simulink model "rover_sw_pwrtrain_24b"  (R2024b)
settings: Solver=FixedStepAuto  StartTime=0.0  StopTime=inf  FixedStep=.01  RelTol=1e-3
values from neighbouring files (symbols this model uses):
  collision_flt : value not decoded    [rover_param.sldd]
  FALSE = 0.0    [rover_param.sldd]
  TRUE = 1.0    [rover_param.sldd]
undefined symbols (not defined in the file or in its folder): DiscIntNeverNeededParam
libraries: ros2lib x36, simulink x5
settings Model: DataDictionary=rover_param.sldd  Creator=abhijeetsaini  LastModifiedBy=saini
settings OptimizationCC: DefaultParameterBehavior=Inlined  EnhancedBackFolding=on  PassReuseOutputArgsThreshold=0  ZeroExternalMemoryAtStartup=off  ZeroInternalMemoryAtStartup=off  MaxStackSize=64  OptimizeBlockOrder=speed  DifferentSizesBufferReuse=on  OptimizationCustomize=off
settings DebuggingCC: ParameterTunabilityLossMsg=error
settings HardwareCC: ProdBitPerLong=64  ProdHWDeviceType=Apple->ARM64  UseEmbeddedCoderFeatures=off
settings RTWCC: Description=Embedded Coder  SystemTargetFile=ert.tlc  HardwareBoard=Robot Operating System 2 (ROS 2)  TLCOptions="-aInlineSetEventsForThisBaseRateFcn=TLC_FALSE -aSuppressMultiTaskScheduler=TLC_FALSE  -aRateBasedStepFcn=0"  TemplateMakefile=ert_default_tmf  Toolchain=Colcon Tools  TargetLang=C++
settings RTWCC: CustomSourceCode=|
  | int  vesc_open_noargs(void);
  | void vesc_close(void);
  | int  vesc_send_duty(double duty);
  | int  vesc_poll(float* v_in, float* t_mos, float* t_motor);
settings CodeAppCC: ForceParamTrailComments=on  OperatorAnnotations=on
settings ERTTargetCC: ERTCustomFileBanners=off  CodeInterfacePackaging=C++ class  SupportContinuousTime=on  SupportNonInlinedSFcns=on  RemoveResetFunc=off  ModelStepFunctionPrototypeControlCompliant=off  RootIOFormat=Structure reference

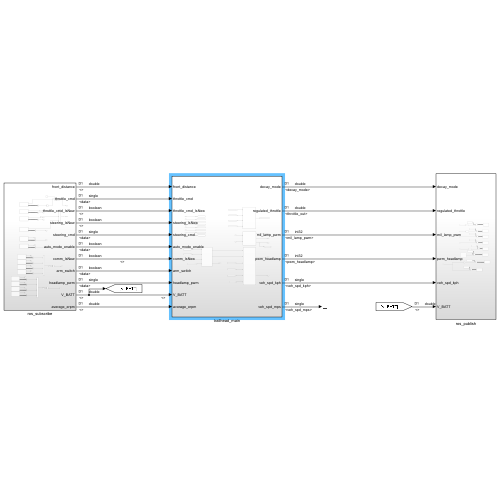
[thumbnail: Simulink's stored preview of the top-level diagram]
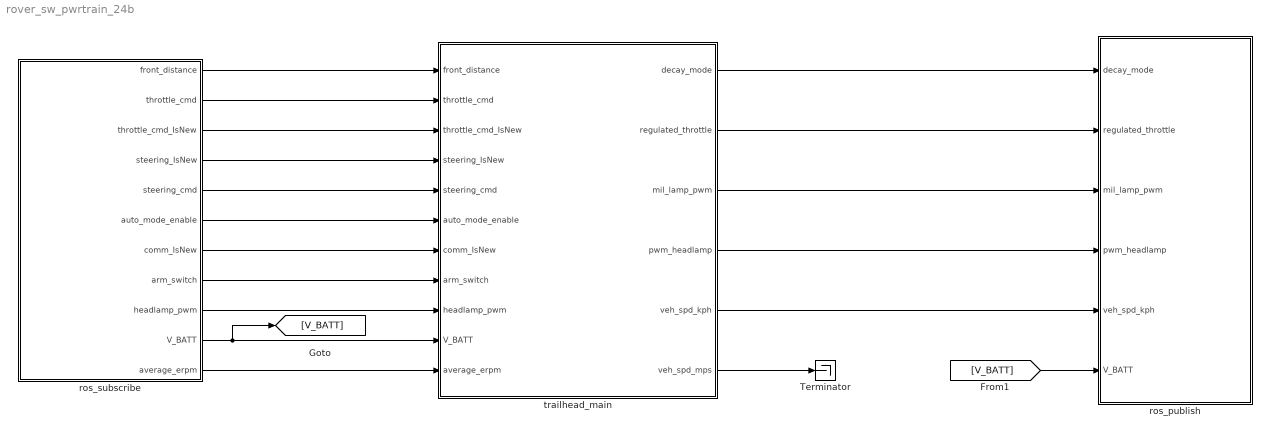
== system rover_sw_pwrtrain_24b ==
  Terminator : Terminator
  ros_publish : Subsystem
  ros_subscribe : Subsystem
  trailhead_main : Subsystem
  wires:
  ros_subscribe/1(front_distance) -> trailhead_main/1(front_distance)
  ros_subscribe/2(throttle_cmd) -> trailhead_main/2(throttle_cmd)
  ros_subscribe/3(throttle_cmd_IsNew) -> trailhead_main/3(throttle_cmd_IsNew)
  ros_subscribe/4(steering_IsNew) -> trailhead_main/4(steering_IsNew)
  ros_subscribe/5(steering_cmd) -> trailhead_main/5(steering_cmd)
  ros_subscribe/7(comm_IsNew) -> trailhead_main/7(comm_IsNew)
  trailhead_main/1(decay_mode) -> ros_publish/1(decay_mode)
  trailhead_main/2(regulated_throttle) -> ros_publish/2(regulated_throttle)
  ros_subscribe/8(arm_switch) -> trailhead_main/8(arm_switch)
  trailhead_main/3(mil_lamp_pwm) -> ros_publish/3(mil_lamp_pwm)
  trailhead_main/4(pwm_headlamp) -> ros_publish/4(pwm_headlamp)
  ros_subscribe/9(headlamp_pwm) -> trailhead_main/9(headlamp_pwm)
  ros_subscribe/10(V_BATT) -> [V_BATT], trailhead_main/10(V_BATT)
  [V_BATT] -> ros_publish/6(V_BATT)
  ros_subscribe/6(auto_mode_enable) -> trailhead_main/6(auto_mode_enable)
  ros_subscribe/11(average_erpm) -> trailhead_main/11(average_erpm)
  trailhead_main/5(veh_spd_kph) -> ros_publish/5(veh_spd_kph)
  trailhead_main/6(veh_spd_mps) -> Terminator/1

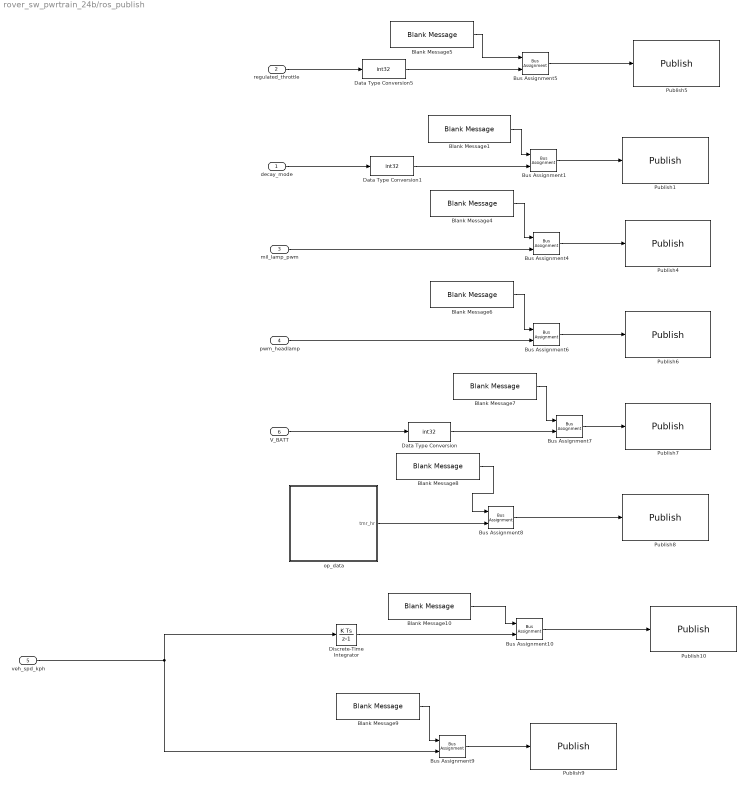
== system rover_sw_pwrtrain_24b/ros_publish ==
  decay_mode : Inport
  regulated_throttle : Inport  Port=2
  mil_lamp_pwm : Inport  Port=3
  pwm_headlamp : Inport  Port=4
  veh_spd_kph : Inport  Port=5
  V_BATT : Inport  Port=6
  Blank Message{1,4..7} (5 alike) : ros2lib/Blank Message  messageClass=Message  entityType=std_msgs/Int32  messageType=std_msgs/Int32  SampleTime=inf
  Blank Message10 : ros2lib/Blank Message  messageClass=Message  entityType=std_msgs/Float32  messageType=std_msgs/Float32  SampleTime=inf
  Blank Message8 : ros2lib/Blank Message  messageClass=Message  entityType=std_msgs/Float32  messageType=std_msgs/Float32  SampleTime=inf
  Blank Message9 : ros2lib/Blank Message  messageClass=Message  entityType=std_msgs/Float32  messageType=std_msgs/Float32  SampleTime=inf
  Bus Assignment{1,4..10} (8 alike) : BusAssignment  AssignedSignals=data
  Data Type Conversion : DataTypeConversion  OutDataTypeStr=int32  SaturateOnIntegerOverflow=off  RndMeth=Floor
  Data Type Conversion1 : DataTypeConversion  OutDataTypeStr=int32  SaturateOnIntegerOverflow=off  RndMeth=Floor
  Data Type Conversion5 : DataTypeConversion  OutDataTypeStr=int32  SaturateOnIntegerOverflow=off  RndMeth=Floor
  Discrete-Time Integrator : DiscreteIntegrator  SampleTime=-1  ICPrevOutput=DiscIntNeverNeededParam  ICPrevScaledInput=DiscIntNeverNeededParam
  Publish1 : ros2lib/Publish  topicSource=Specify your own  topic=/decay_mode  messageType=std_msgs/Int32  QOSHistory=Keep last  QOSDepth=1  QOSReliability=Reliable  QOSDurability=Volatile  QOSDeadline=Inf  QOSLifespan=Inf  QOSLiveliness=Automatic  QOSLeaseDuration=Inf  QOSAvoidROSNamespaceConventions=off
  Publish10 : ros2lib/Publish  topicSource=Specify your own  topic=/stats/distance  messageType=std_msgs/Float32  QOSHistory=Keep last  QOSDepth=1  QOSReliability=Reliable  QOSDurability=Volatile  QOSDeadline=Inf  QOSLifespan=Inf  QOSLiveliness=Automatic  QOSLeaseDuration=Inf  QOSAvoidROSNamespaceConventions=off
  Publish4 : ros2lib/Publish  topicSource=Specify your own  topic=/pwm/mil  messageType=std_msgs/Int32  QOSHistory=Keep last  QOSDepth=1  QOSReliability=Reliable  QOSDurability=Volatile  QOSDeadline=Inf  QOSLifespan=Inf  QOSLiveliness=Automatic  QOSLeaseDuration=Inf  QOSAvoidROSNamespaceConventions=off
  Publish5 : ros2lib/Publish  topicSource=Specify your own  topic=/throttel_regulated  messageType=std_msgs/Int32  QOSHistory=Keep last  QOSDepth=1  QOSReliability=Reliable  QOSDurability=Volatile  QOSDeadline=Inf  QOSLifespan=Inf  QOSLiveliness=Automatic  QOSLeaseDuration=Inf  QOSAvoidROSNamespaceConventions=off
  Publish6 : ros2lib/Publish  topicSource=Specify your own  topic=/pwm/headlamp  messageType=std_msgs/Int32  QOSHistory=Keep last  QOSDepth=1  QOSReliability=Reliable  QOSDurability=Volatile  QOSDeadline=Inf  QOSLifespan=Inf  QOSLiveliness=Automatic  QOSLeaseDuration=Inf  QOSAvoidROSNamespaceConventions=off
  Publish7 : ros2lib/Publish  topicSource=Specify your own  topic=v_batt_av  messageType=std_msgs/Int32  QOSHistory=Keep last  QOSDepth=1  QOSReliability=Reliable  QOSDurability=Volatile  QOSDeadline=Inf  QOSLifespan=Inf  QOSLiveliness=Automatic  QOSLeaseDuration=Inf  QOSAvoidROSNamespaceConventions=off
  Publish8 : ros2lib/Publish  topicSource=Specify your own  topic=/stats/op_hours  messageType=std_msgs/Float32  QOSHistory=Keep last  QOSDepth=1  QOSReliability=Reliable  QOSDurability=Volatile  QOSDeadline=Inf  QOSLifespan=Inf  QOSLiveliness=Automatic  QOSLeaseDuration=Inf  QOSAvoidROSNamespaceConventions=off
  Publish9 : ros2lib/Publish  topicSource=Specify your own  topic=/stats/avg_speed  messageType=std_msgs/Float32  QOSHistory=Keep last  QOSDepth=1  QOSReliability=Reliable  QOSDurability=Volatile  QOSDeadline=Inf  QOSLifespan=Inf  QOSLiveliness=Automatic  QOSLeaseDuration=Inf  QOSAvoidROSNamespaceConventions=off
  op_data : Stateflow chart  TreatAsAtomicUnit=on
  wires:
  Bus Assignment5/1 -> Publish5/1
  Data Type Conversion5/1 -> Bus Assignment5/2
  Blank Message5/1 -> Bus Assignment5/1
  regulated_throttle/1 -> Data Type Conversion5/1
  Data Type Conversion1/1 -> Bus Assignment1/2
  Bus Assignment1/1 -> Publish1/1
  decay_mode/1 -> Data Type Conversion1/1
  Blank Message1/1 -> Bus Assignment1/1
  mil_lamp_pwm/1 -> Bus Assignment4/2
  Bus Assignment4/1 -> Publish4/1
  Blank Message4/1 -> Bus Assignment4/1
  pwm_headlamp/1 -> Bus Assignment6/2
  Blank Message6/1 -> Bus Assignment6/1
  Bus Assignment6/1 -> Publish6/1
  Bus Assignment7/1 -> Publish7/1
  V_BATT/1 -> Data Type Conversion/1
  Blank Message7/1 -> Bus Assignment7/1
  Data Type Conversion/1 -> Bus Assignment7/2
  Bus Assignment8/1 -> Publish8/1
  Blank Message8/1 -> Bus Assignment8/1
  Bus Assignment9/1 -> Publish9/1
  Blank Message9/1 -> Bus Assignment9/1
  veh_spd_kph/1 -> Discrete-Time Integrator/1, Bus Assignment9/2
  op_data/1(tmr_hr) -> Bus Assignment8/2
  Discrete-Time Integrator/1 -> Bus Assignment10/2
  Blank Message10/1 -> Bus Assignment10/1
  Bus Assignment10/1 -> Publish10/1

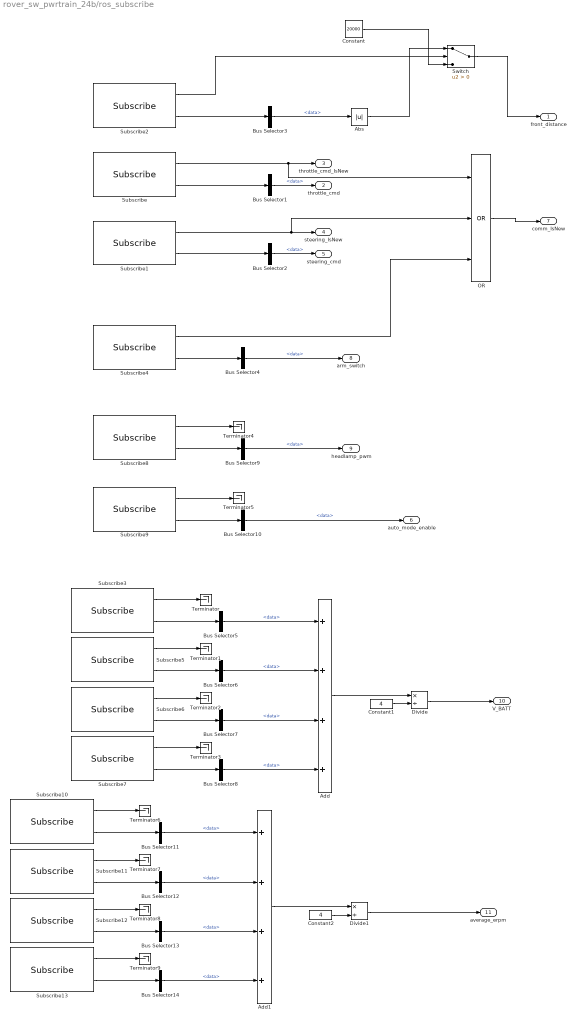
== system rover_sw_pwrtrain_24b/ros_subscribe ==
  Abs : Abs  SaturateOnIntegerOverflow=off
  Add : Sum  Inputs=++++
  Add1 : Sum  Inputs=++++
  Bus Selector{1..14} (14 alike) : BusSelector  OutputSignals=data
  Constant : Constant  Value=20000
  Constant1 : Constant  Value=4
  Constant2 : Constant  Value=4
  Divide : Product  Inputs=*/
  Divide1 : Product  Inputs=*/
  OR : Logic  Operator=OR  Inputs=3  AllPortsSameDT=off  OutDataTypeStr=boolean
  Subscribe : ros2lib/Subscribe  topicSource=Specify your own  topic=/rc/ch1  messageType=std_msgs/Float32  sampleTime=-1  QOSHistory=Keep last  QOSDepth=1  QOSReliability=Reliable  QOSDurability=Volatile  QOSDeadline=Inf  QOSLifespan=Inf  QOSLiveliness=Automatic  QOSLeaseDuration=Inf  QOSAvoidROSNamespaceConventions=off
  Subscribe1 : ros2lib/Subscribe  topicSource=Specify your own  topic=/rc/ch2  messageType=std_msgs/Float32  sampleTime=-1  QOSHistory=Keep last  QOSDepth=1  QOSReliability=Reliable  QOSDurability=Volatile  QOSDeadline=Inf  QOSLifespan=Inf  QOSLiveliness=Automatic  QOSLeaseDuration=Inf  QOSAvoidROSNamespaceConventions=off
  Subscribe10 : ros2lib/Subscribe  topicSource=Specify your own  topic=/vesc/rpm/rf  messageType=std_msgs/Float32  sampleTime=-1  QOSHistory=Keep last  QOSDepth=1  QOSReliability=Reliable  QOSDurability=Volatile  QOSDeadline=Inf  QOSLifespan=Inf  QOSLiveliness=Automatic  QOSLeaseDuration=Inf  QOSAvoidROSNamespaceConventions=off
  Subscribe11 : ros2lib/Subscribe  topicSource=Specify your own  topic=/vesc/rpm/lr  messageType=std_msgs/Float32  sampleTime=-1  QOSHistory=Keep last  QOSDepth=1  QOSReliability=Reliable  QOSDurability=Volatile  QOSDeadline=Inf  QOSLifespan=Inf  QOSLiveliness=Automatic  QOSLeaseDuration=Inf  QOSAvoidROSNamespaceConventions=off
  Subscribe12 : ros2lib/Subscribe  topicSource=Specify your own  topic=/vesc/rpm/rf  messageType=std_msgs/Float32  sampleTime=-1  QOSHistory=Keep last  QOSDepth=1  QOSReliability=Reliable  QOSDurability=Volatile  QOSDeadline=Inf  QOSLifespan=Inf  QOSLiveliness=Automatic  QOSLeaseDuration=Inf  QOSAvoidROSNamespaceConventions=off
  Subscribe13 : ros2lib/Subscribe  topicSource=Specify your own  topic=/vesc/rpm/rr  messageType=std_msgs/Float32  sampleTime=-1  QOSHistory=Keep last  QOSDepth=1  QOSReliability=Reliable  QOSDurability=Volatile  QOSDeadline=Inf  QOSLifespan=Inf  QOSLiveliness=Automatic  QOSLeaseDuration=Inf  QOSAvoidROSNamespaceConventions=off
  Subscribe2 : ros2lib/Subscribe  topicSource=Specify your own  topic=/front_distance  messageType=std_msgs/Float32  sampleTime=-1  QOSHistory=Keep last  QOSDepth=1  QOSReliability=Reliable  QOSDurability=Volatile  QOSDeadline=Inf  QOSLifespan=Inf  QOSLiveliness=Automatic  QOSLeaseDuration=Inf  QOSAvoidROSNamespaceConventions=off
  Subscribe3 : ros2lib/Subscribe  topicSource=Specify your own  topic=/vesc/voltage/lf  messageType=std_msgs/Float32  sampleTime=-1  QOSHistory=Keep last  QOSDepth=1  QOSReliability=Reliable  QOSDurability=Volatile  QOSDeadline=Inf  QOSLifespan=Inf  QOSLiveliness=Automatic  QOSLeaseDuration=Inf  QOSAvoidROSNamespaceConventions=off
  Subscribe4 : ros2lib/Subscribe  topicSource=Specify your own  topic=/rc/ch3  messageType=std_msgs/Bool  sampleTime=-1  QOSHistory=Keep last  QOSDepth=1  QOSReliability=Reliable  QOSDurability=Volatile  QOSDeadline=Inf  QOSLifespan=Inf  QOSLiveliness=Automatic  QOSLeaseDuration=Inf  QOSAvoidROSNamespaceConventions=off
  Subscribe5 : ros2lib/Subscribe  topicSource=Specify your own  topic=/vesc/voltage/lr  messageType=std_msgs/Float32  sampleTime=-1  QOSHistory=Keep last  QOSDepth=1  QOSReliability=Reliable  QOSDurability=Volatile  QOSDeadline=Inf  QOSLifespan=Inf  QOSLiveliness=Automatic  QOSLeaseDuration=Inf  QOSAvoidROSNamespaceConventions=off
  Subscribe6 : ros2lib/Subscribe  topicSource=Specify your own  topic=/vesc/voltage/rf  messageType=std_msgs/Float32  sampleTime=-1  QOSHistory=Keep last  QOSDepth=1  QOSReliability=Reliable  QOSDurability=Volatile  QOSDeadline=Inf  QOSLifespan=Inf  QOSLiveliness=Automatic  QOSLeaseDuration=Inf  QOSAvoidROSNamespaceConventions=off
  Subscribe7 : ros2lib/Subscribe  topicSource=Specify your own  topic=/vesc/voltage/rr  messageType=std_msgs/Float32  sampleTime=-1  QOSHistory=Keep last  QOSDepth=1  QOSReliability=Reliable  QOSDurability=Volatile  QOSDeadline=Inf  QOSLifespan=Inf  QOSLiveliness=Automatic  QOSLeaseDuration=Inf  QOSAvoidROSNamespaceConventions=off
  Subscribe8 : ros2lib/Subscribe  topicSource=Specify your own  topic=/rc/ch4  messageType=std_msgs/Float32  sampleTime=-1  QOSHistory=Keep last  QOSDepth=1  QOSReliability=Reliable  QOSDurability=Volatile  QOSDeadline=Inf  QOSLifespan=Inf  QOSLiveliness=Automatic  QOSLeaseDuration=Inf  QOSAvoidROSNamespaceConventions=off
  Subscribe9 : ros2lib/Subscribe  topicSource=Specify your own  topic=/rc/ch7  messageType=std_msgs/Bool  sampleTime=-1  QOSHistory=Keep last  QOSDepth=1  QOSReliability=Reliable  QOSDurability=Volatile  QOSDeadline=Inf  QOSLifespan=Inf  QOSLiveliness=Automatic  QOSLeaseDuration=Inf  QOSAvoidROSNamespaceConventions=off
  Switch : Switch  Criteria=u2 > Threshold  SaturateOnIntegerOverflow=off  InputSameDT=off
  Terminator{,1..9} (10 alike) : Terminator
  front_distance : Outport
  throttle_cmd : Outport  Port=2
  throttle_cmd_IsNew : Outport  Port=3
  steering_IsNew : Outport  Port=4
  steering_cmd : Outport  Port=5
  auto_mode_enable : Outport  Port=6
  comm_IsNew : Outport  Port=7
  arm_switch : Outport  Port=8
  headlamp_pwm : Outport  Port=9
  V_BATT : Outport  Port=10
  average_erpm : Outport  Port=11
  wires:
  Subscribe2/2 -> Bus Selector3/1
  Subscribe1/2 -> Bus Selector2/1
  Subscribe/2 -> Bus Selector1/1
  Bus Selector3/1 -> Abs/1  "<data>"
  Subscribe2/1 -> Switch/2
  Bus Selector1/1 -> throttle_cmd/1  "<data>"
  Subscribe/1 -> throttle_cmd_IsNew/1, OR/1
  Subscribe1/1 -> OR/2, steering_IsNew/1
  Bus Selector2/1 -> steering_cmd/1  "<data>"
  Abs/1 -> Switch/1
  OR/1 -> comm_IsNew/1
  Constant/1 -> Switch/3
  Switch/1 -> front_distance/1
  Subscribe4/1 -> OR/3
  Subscribe4/2 -> Bus Selector4/1
  Bus Selector4/1 -> arm_switch/1  "<data>"
  Bus Selector5/1 -> Add/1  "<data>"
  Subscribe3/2 -> Bus Selector5/1
  Bus Selector6/1 -> Add/2  "<data>"
  Subscribe5/2 -> Bus Selector6/1
  Bus Selector7/1 -> Add/3  "<data>"
  Subscribe6/2 -> Bus Selector7/1
  Bus Selector8/1 -> Add/4  "<data>"
  Subscribe7/2 -> Bus Selector8/1
  Add/1 -> Divide/1
  Constant1/1 -> Divide/2
  Divide/1 -> V_BATT/1
  Subscribe3/1 -> Terminator/1
  Subscribe5/1 -> Terminator1/1
  Subscribe6/1 -> Terminator2/1
  Subscribe7/1 -> Terminator3/1
  Bus Selector9/1 -> headlamp_pwm/1  "<data>"
  Subscribe8/2 -> Bus Selector9/1
  Subscribe8/1 -> Terminator4/1
  Subscribe9/1 -> Terminator5/1
  Subscribe9/2 -> Bus Selector10/1
  Bus Selector10/1 -> auto_mode_enable/1  "<data>"
  Subscribe10/2 -> Bus Selector11/1
  Subscribe13/1 -> Terminator9/1
  Divide1/1 -> average_erpm/1
  Subscribe12/1 -> Terminator8/1
  Add1/1 -> Divide1/1
  Bus Selector13/1 -> Add1/3  "<data>"
  Bus Selector11/1 -> Add1/1  "<data>"
  Bus Selector12/1 -> Add1/2  "<data>"
  Subscribe11/1 -> Terminator7/1
  Bus Selector14/1 -> Add1/4  "<data>"
  Subscribe11/2 -> Bus Selector12/1
  Constant2/1 -> Divide1/2
  Subscribe13/2 -> Bus Selector14/1
  Subscribe10/1 -> Terminator6/1
  Subscribe12/2 -> Bus Selector13/1

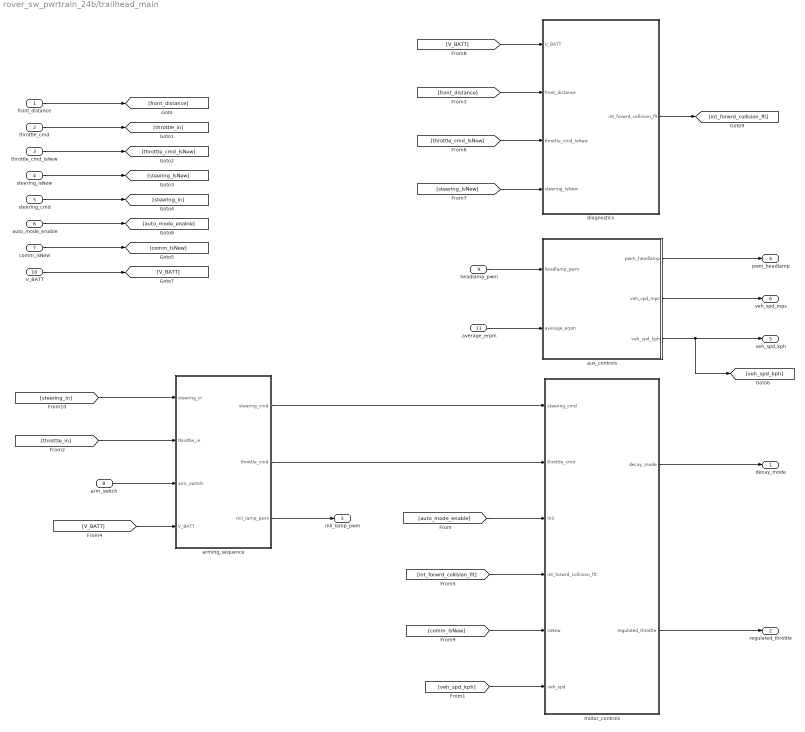
== system rover_sw_pwrtrain_24b/trailhead_main ==
  front_distance : Inport
  throttle_cmd : Inport  Port=2
  throttle_cmd_IsNew : Inport  Port=3
  steering_IsNew : Inport  Port=4
  steering_cmd : Inport  Port=5
  auto_mode_enable : Inport  Port=6
  comm_IsNew : Inport  Port=7
  arm_switch : Inport  Port=8
  headlamp_pwm : Inport  Port=9
  V_BATT : Inport  Port=10
  average_erpm : Inport  Port=11
  arming_sequence : Subsystem
  aux_controls : Subsystem
  diagnostics : Subsystem
  motor_controls : Subsystem
  decay_mode : Outport
  regulated_throttle : Outport  Port=2
  mil_lamp_pwm : Outport  Port=3
  pwm_headlamp : Outport  Port=4
  veh_spd_kph : Outport  Port=5
  veh_spd_mps : Outport  Port=6
  wires:
  motor_controls/2(regulated_throttle) -> regulated_throttle/1
  front_distance/1 -> [front_distance]
  [comm_IsNew] -> motor_controls/5(IsNew)
  motor_controls/1(decay_mode) -> decay_mode/1
  throttle_cmd_IsNew/1 -> [throttle_cmd_IsNew]
  comm_IsNew/1 -> [comm_IsNew]
  [int_forwrd_collision_flt] -> motor_controls/4(int_forwrd_collision_flt)
  [throttle_cmd_IsNew] -> diagnostics/3(throttle_cmd_IsNew)
  steering_cmd/1 -> [steering_in]
  diagnostics/1(int_forwrd_collision_flt) -> [int_forwrd_collision_flt]
  [steering_in] -> arming_sequence/1(steering_in)
  steering_IsNew/1 -> [steering_IsNew]
  auto_mode_enable/1 -> [auto_mode_enable]
  [front_distance] -> diagnostics/2(front_distance)
  [throttle_in] -> arming_sequence/2(throttle_in)
  arming_sequence/1(steering_cmd) -> motor_controls/1(steering_cmd)
  throttle_cmd/1 -> [throttle_in]
  [steering_IsNew] -> diagnostics/4(steering_IsNew)
  arming_sequence/2(throttle_cmd) -> motor_controls/2(throttle_cmd)
  arm_switch/1 -> arming_sequence/3(arm_switch)
  V_BATT/1 -> [V_BATT]
  arming_sequence/3(mil_lamp_pwm) -> mil_lamp_pwm/1
  aux_controls/1(pwm_headlamp) -> pwm_headlamp/1
  headlamp_pwm/1 -> aux_controls/1(headlamp_pwm)
  [auto_mode_enable] -> motor_controls/3(In3)
  average_erpm/1 -> aux_controls/2(average_erpm)
  aux_controls/2(veh_spd_mps) -> veh_spd_mps/1
  aux_controls/3(veh_spd_kph) -> veh_spd_kph/1, [veh_spd_kph]
  [veh_spd_kph] -> motor_controls/6(veh_spd)
  [V_BATT] -> arming_sequence/4(V_BATT)
  [V_BATT] -> diagnostics/1(V_BATT)

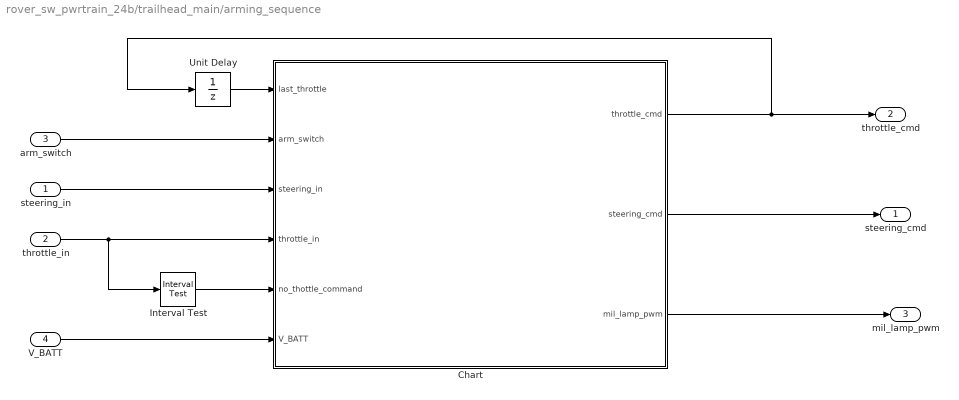
== system rover_sw_pwrtrain_24b/trailhead_main/arming_sequence ==
  steering_in : Inport
  throttle_in : Inport  Port=2
  arm_switch : Inport  Port=3
  V_BATT : Inport  Port=4
  Chart : Stateflow chart  TreatAsAtomicUnit=on
      settings: PortSchema="{\"entries\":[{\"content\":{\"sides\":[{\"content\":{\"connectorIds\":[\"In1\",\"In4\",\"In2\",\"In3\",\"In5\",\"In6\"]},\"type\":\"ConnectorPlacement.EquallySpacedRectSide\",\"uuid\":\"c108e5ce-30df-4295-bedd-99ebe70d8a91\"},{\"content\":{\"connectorIds\":[\"Out1\",\"Out3\",\"Out2\"],\"side\":\"RIGHT\"},\"type\":\"ConnectorPlacement.EquallySpacedRectSide\",\"uuid\":\"b8e5dff0-21b7-4fab-bebb-64376f336a1d\"},{\"content\":{\"side\":\"TOP\"},\"type\":\"ConnectorPlacement.EquallySpacedRectSide\",\"uuid\":\"eff58cc0-4cc9-4f0b-b377-20fc9f00e10d\"}]},\"type\":\"ConnectorPlacement.EquallySpacedConnector\",\"uuid\":\"fbbe158e-b65f-47b7-ae26-4517c910f89e\"}],\"packageUris\":[\"http://schema.mathworks.com/mf0/Connector/R2020b\"],\"version\":\"1.0\"}"
  Interval Test : simulink/Logic and Bit Operations/Interval Test  IntervalClosedRight=on  uplimit=.1  IntervalClosedLeft=on  lowlimit=-.1  OutDataTypeStr=boolean
  Unit Delay : UnitDelay  SampleTime=-1  HasFrameUpgradeWarning=on
  steering_cmd : Outport
  throttle_cmd : Outport  Port=2
  mil_lamp_pwm : Outport  Port=3
  wires:
  throttle_in/1 -> Interval Test/1, Chart/3(throttle_in)
  steering_in/1 -> Chart/2(steering_in)
  arm_switch/1 -> Chart/4(arm_switch)
  V_BATT/1 -> Chart/6(V_BATT)
  Chart/3(steering_cmd) -> steering_cmd/1
  Chart/1(throttle_cmd) -> Unit Delay/1, throttle_cmd/1
  Chart/2(mil_lamp_pwm) -> mil_lamp_pwm/1
  Interval Test/1 -> Chart/5(no_thottle_command)
  Unit Delay/1 -> Chart/1(last_throttle)

== system rover_sw_pwrtrain_24b/trailhead_main/aux_controls ==
  headlamp_pwm : Inport
  average_erpm : Inport  Port=2
  Subsystem : Subsystem
  Subsystem1 : Subsystem
  pwm_headlamp : Outport
  veh_spd_mps : Outport  Port=2
  veh_spd_kph : Outport  Port=3
  wires:
  headlamp_pwm/1 -> Subsystem/1(headlamp_pwm)
  Subsystem/1(pwm_headlamp) -> pwm_headlamp/1
  average_erpm/1 -> Subsystem1/1(average_erpm)
  Subsystem1/1(veh_spd_mps) -> veh_spd_mps/1
  Subsystem1/2(veh_spd_kph) -> veh_spd_kph/1

== system rover_sw_pwrtrain_24b/trailhead_main/diagnostics ==
  V_BATT : Inport
  front_distance : Inport  Port=2
  throttle_cmd_IsNew : Inport  Port=3
  steering_IsNew : Inport  Port=4
  Subsystem : Subsystem
  int_forwrd_collision_flt : Outport
  wires:
  front_distance/1 -> Subsystem/1(front_distance)
  Subsystem/1(int_forwrd_collision_flt) -> int_forwrd_collision_flt/1
  V_BATT/1 -> ?

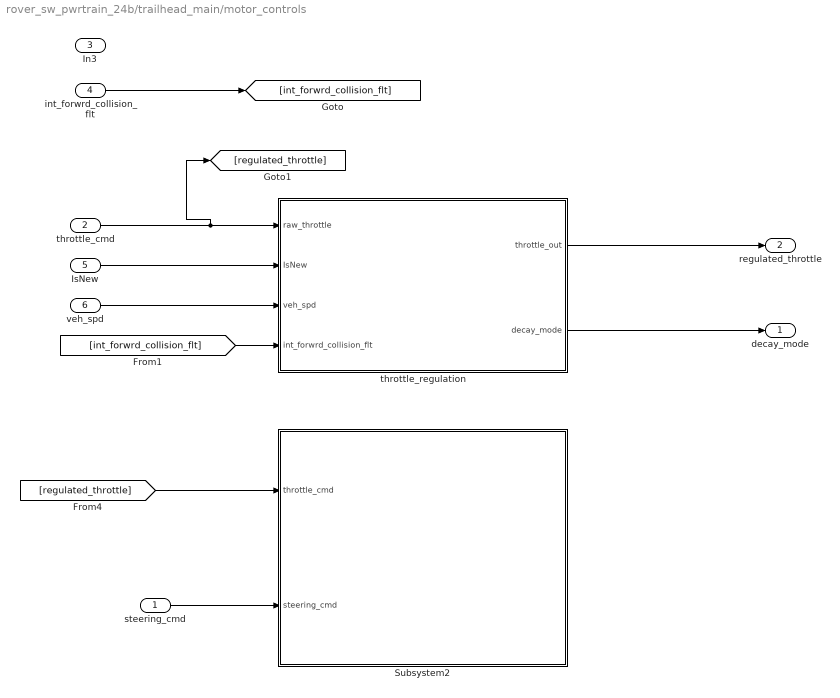
== system rover_sw_pwrtrain_24b/trailhead_main/motor_controls ==
  steering_cmd : Inport
  throttle_cmd : Inport  Port=2
  In3 : Inport  Port=3
  int_forwrd_collision_flt : Inport  Port=4
  IsNew : Inport  Port=5
  veh_spd : Inport  Port=6
  Subsystem2 : Subsystem
  throttle_regulation : Subsystem
  decay_mode : Outport
  regulated_throttle : Outport  Port=2
  wires:
  throttle_cmd/1 -> [regulated_throttle], throttle_regulation/1(raw_throttle)
  steering_cmd/1 -> Subsystem2/2(steering_cmd)
  IsNew/1 -> throttle_regulation/2(IsNew)
  throttle_regulation/2(decay_mode) -> decay_mode/1
  throttle_regulation/1(throttle_out) -> regulated_throttle/1
  veh_spd/1 -> throttle_regulation/3(veh_spd)
  int_forwrd_collision_flt/1 -> [int_forwrd_collision_flt]
  [int_forwrd_collision_flt] -> throttle_regulation/4(int_forwrd_collision_flt)
  [regulated_throttle] -> Subsystem2/1(throttle_cmd)

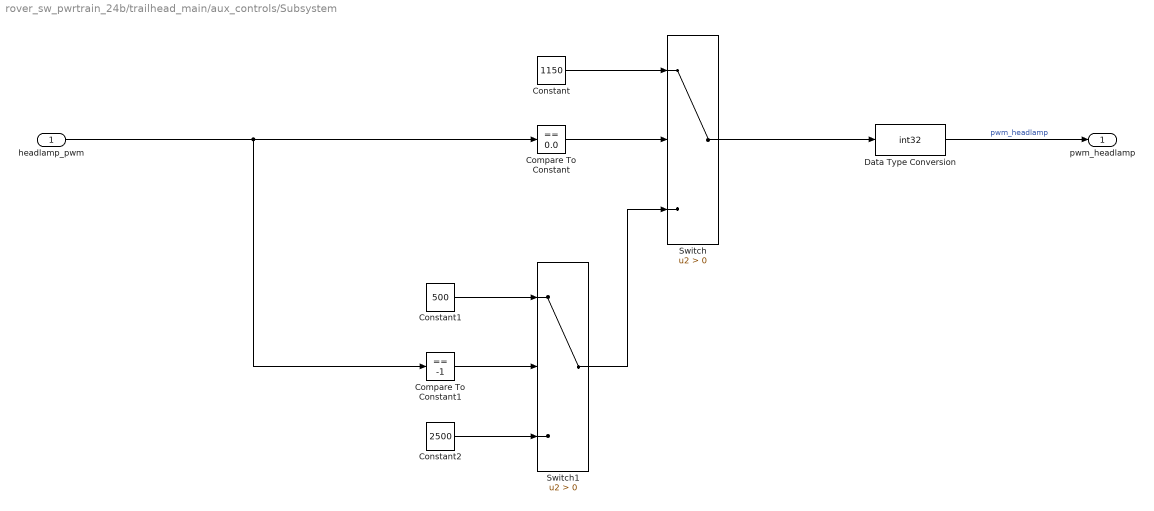
== system rover_sw_pwrtrain_24b/trailhead_main/aux_controls/Subsystem ==
  headlamp_pwm : Inport
  Compare To Constant : simulink/Logic and Bit Operations/Compare To Constant  relop===  const=0.0  OutDataTypeStr=boolean
  Compare To Constant1 : simulink/Logic and Bit Operations/Compare To Constant  relop===  const=-1  OutDataTypeStr=boolean
  Constant : Constant  Value=1150
  Constant1 : Constant  Value=500
  Constant2 : Constant  Value=2500
  Data Type Conversion : DataTypeConversion  OutDataTypeStr=int32  SaturateOnIntegerOverflow=off  RndMeth=Floor
  Switch : Switch  Criteria=u2 > Threshold  SaturateOnIntegerOverflow=off  InputSameDT=off
  Switch1 : Switch  Criteria=u2 > Threshold  SaturateOnIntegerOverflow=off  InputSameDT=off
  pwm_headlamp : Outport
  wires:
  headlamp_pwm/1 -> Compare To Constant1/1, Compare To Constant/1
  Compare To Constant/1 -> Switch/2
  Constant/1 -> Switch/1
  Compare To Constant1/1 -> Switch1/2
  Constant1/1 -> Switch1/1
  Constant2/1 -> Switch1/3
  Switch1/1 -> Switch/3
  Switch/1 -> Data Type Conversion/1
  Data Type Conversion/1 -> pwm_headlamp/1  "pwm_headlamp"

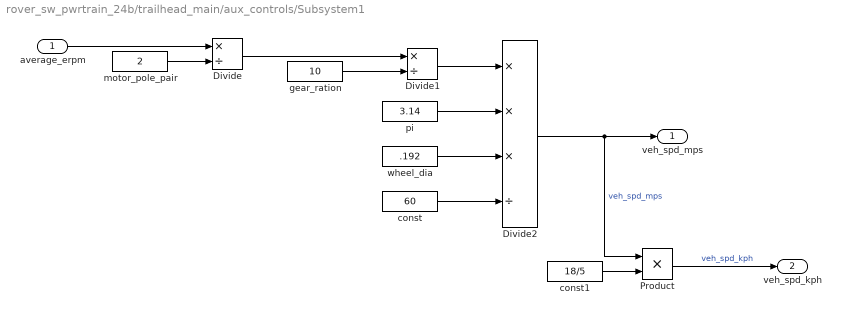
== system rover_sw_pwrtrain_24b/trailhead_main/aux_controls/Subsystem1 ==
  average_erpm : Inport
  Divide : Product  Inputs=*/
  Divide1 : Product  Inputs=*/
  Divide2 : Product  Inputs=***/  OutDataTypeStr=single
  Product : Product  OutDataTypeStr=single
  const : Constant  Value=60
  const1 : Constant  Value=18/5
  gear_ration : Constant  Value=10
  motor_pole_pair : Constant  Value=2
  pi : Constant  Value=3.14
  wheel_dia : Constant  Value=.192
  veh_spd_mps : Outport
  veh_spd_kph : Outport  Port=2
  wires:
  average_erpm/1 -> Divide/1
  motor_pole_pair/1 -> Divide/2
  Divide/1 -> Divide1/1
  gear_ration/1 -> Divide1/2
  Divide1/1 -> Divide2/1
  pi/1 -> Divide2/2
  wheel_dia/1 -> Divide2/3
  const/1 -> Divide2/4
  Divide2/1 -> Product/1, veh_spd_mps/1  "veh_spd_mps"
  Product/1 -> veh_spd_kph/1  "veh_spd_kph"
  const1/1 -> Product/2

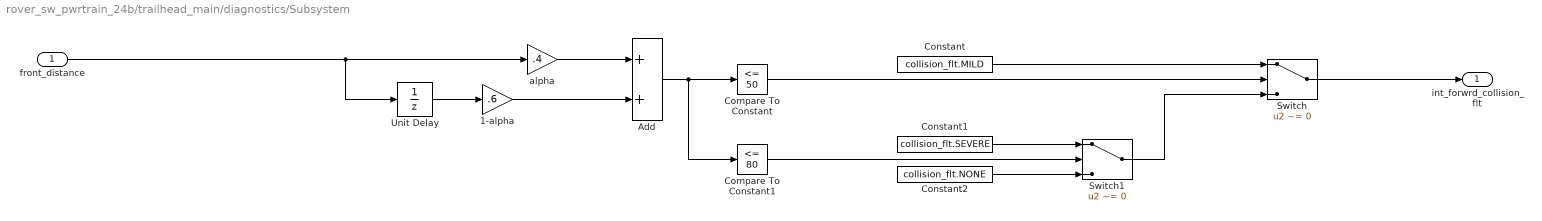
== system rover_sw_pwrtrain_24b/trailhead_main/diagnostics/Subsystem ==
  front_distance : Inport
  1-alpha : Gain  Gain=.6
  Add : Sum
  Compare To Constant : simulink/Logic and Bit Operations/Compare To Constant  relop=<=  const=50  OutDataTypeStr=boolean
  Compare To Constant1 : simulink/Logic and Bit Operations/Compare To Constant  relop=<=  const=80  OutDataTypeStr=boolean
  Constant : Constant  Value=collision_flt.MILD
  Constant1 : Constant  Value=collision_flt.SEVERE
  Constant2 : Constant  Value=collision_flt.NONE
  Switch : Switch  Criteria=u2 ~= 0  SaturateOnIntegerOverflow=off  InputSameDT=off
  Switch1 : Switch  Criteria=u2 ~= 0  SaturateOnIntegerOverflow=off  InputSameDT=off
  Unit Delay : UnitDelay  SampleTime=-1  HasFrameUpgradeWarning=on
  alpha : Gain  Gain=.4
  int_forwrd_collision_flt : Outport
  wires:
  Switch/1 -> int_forwrd_collision_flt/1
  Constant2/1 -> Switch1/3
  Compare To Constant/1 -> Switch/2
  Switch1/1 -> Switch/3
  Add/1 -> Compare To Constant1/1, Compare To Constant/1
  Constant1/1 -> Switch1/1
  front_distance/1 -> Unit Delay/1, alpha/1
  Compare To Constant1/1 -> Switch1/2
  Constant/1 -> Switch/1
  alpha/1 -> Add/1
  1-alpha/1 -> Add/2
  Unit Delay/1 -> 1-alpha/1

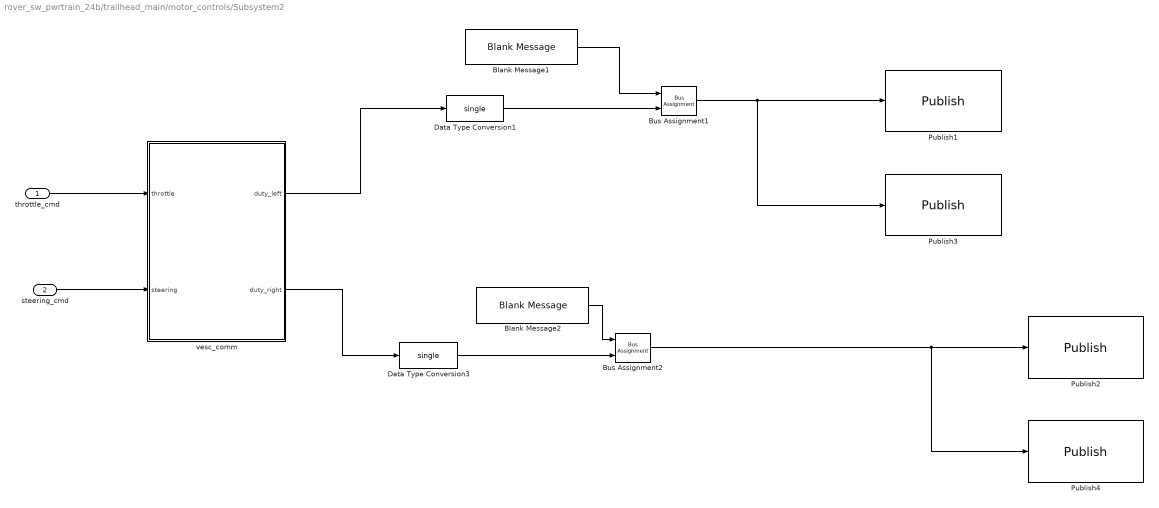
== system rover_sw_pwrtrain_24b/trailhead_main/motor_controls/Subsystem2 ==
  throttle_cmd : Inport
  steering_cmd : Inport  Port=2
  Blank Message1 : ros2lib/Blank Message  messageClass=Message  entityType=std_msgs/Float32  messageType=std_msgs/Float32  SampleTime=inf
  Blank Message2 : ros2lib/Blank Message  messageClass=Message  entityType=std_msgs/Float32  messageType=std_msgs/Float32  SampleTime=inf
  Bus Assignment1 : BusAssignment  AssignedSignals=data
  Bus Assignment2 : BusAssignment  AssignedSignals=data
  Data Type Conversion1 : DataTypeConversion  OutDataTypeStr=single  SaturateOnIntegerOverflow=off  RndMeth=Floor
  Data Type Conversion3 : DataTypeConversion  OutDataTypeStr=single  SaturateOnIntegerOverflow=off  RndMeth=Floor
  Publish1 : ros2lib/Publish  topicSource=Specify your own  topic=/duty/lf  messageType=std_msgs/Float32  QOSHistory=Keep last  QOSDepth=1  QOSReliability=Reliable  QOSDurability=Volatile  QOSDeadline=Inf  QOSLifespan=Inf  QOSLiveliness=Automatic  QOSLeaseDuration=Inf  QOSAvoidROSNamespaceConventions=off
      settings: AttributesFormatString=%<DataTypeOverride_Compiled>
  Publish2 : ros2lib/Publish  topicSource=Specify your own  topic=/duty/rf  messageType=std_msgs/Float32  QOSHistory=Keep last  QOSDepth=1  QOSReliability=Reliable  QOSDurability=Volatile  QOSDeadline=Inf  QOSLifespan=Inf  QOSLiveliness=Automatic  QOSLeaseDuration=Inf  QOSAvoidROSNamespaceConventions=off
  Publish3 : ros2lib/Publish  topicSource=Specify your own  topic=/duty/lr  messageType=std_msgs/Float32  QOSHistory=Keep last  QOSDepth=1  QOSReliability=Reliable  QOSDurability=Volatile  QOSDeadline=Inf  QOSLifespan=Inf  QOSLiveliness=Automatic  QOSLeaseDuration=Inf  QOSAvoidROSNamespaceConventions=off
  Publish4 : ros2lib/Publish  topicSource=Specify your own  topic=/duty/rr  messageType=std_msgs/Float32  QOSHistory=Keep last  QOSDepth=1  QOSReliability=Reliable  QOSDurability=Volatile  QOSDeadline=Inf  QOSLifespan=Inf  QOSLiveliness=Automatic  QOSLeaseDuration=Inf  QOSAvoidROSNamespaceConventions=off
  vesc_comm : Subsystem
  wires:
  vesc_comm/1(duty_left) -> Data Type Conversion1/1
  Bus Assignment1/1 -> Publish3/1, Publish1/1
  steering_cmd/1 -> vesc_comm/2(steering)
  Blank Message1/1 -> Bus Assignment1/1
  vesc_comm/2(duty_right) -> Data Type Conversion3/1
  Data Type Conversion1/1 -> Bus Assignment1/2
  Blank Message2/1 -> Bus Assignment2/1
  throttle_cmd/1 -> vesc_comm/1(throttle)
  Data Type Conversion3/1 -> Bus Assignment2/2
  Bus Assignment2/1 -> Publish2/1, Publish4/1

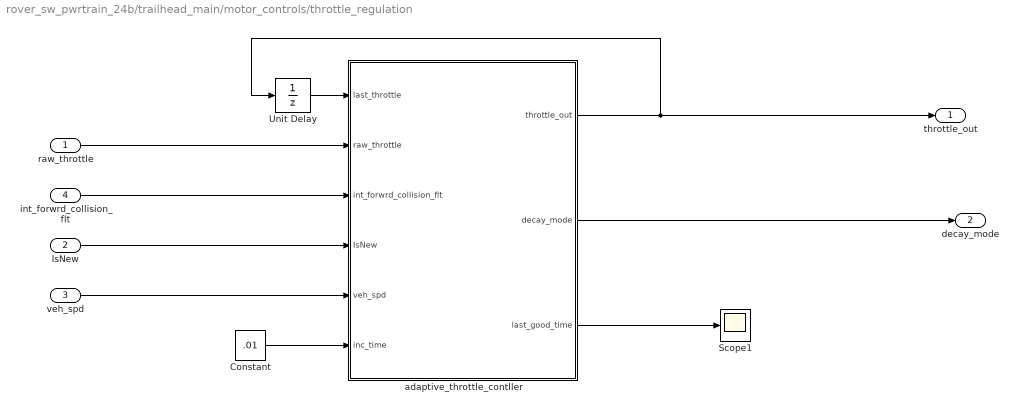
== system rover_sw_pwrtrain_24b/trailhead_main/motor_controls/throttle_regulation ==
  raw_throttle : Inport
  IsNew : Inport  Port=2
  veh_spd : Inport  Port=3
  int_forwrd_collision_flt : Inport  Port=4
  Constant : Constant  Value=.01
  Scope1 : Scope
  Unit Delay : UnitDelay  SampleTime=-1  HasFrameUpgradeWarning=on
  adaptive_throttle_contller : Stateflow chart  TreatAsAtomicUnit=on
      settings: PortSchema="{\"entries\":[{\"content\":{\"sides\":[{\"content\":{\"connectorIds\":[\"In6\",\"In1\",\"In2\",\"In4\",\"In5\",\"In3\"]},\"type\":\"ConnectorPlacement.EquallySpacedRectSide\",\"uuid\":\"a901601a-93d8-4204-afbc-6902d68e8e0d\"},{\"content\":{\"connectorIds\":[\"Out1\",\"Out2\",\"Out3\"],\"side\":\"RIGHT\"},\"type\":\"ConnectorPlacement.EquallySpacedRectSide\",\"uuid\":\"1b6da7a7-1794-4447-8554-df420924e9ae\"},{\"content\":{\"side\":\"TOP\"},\"type\":\"ConnectorPlacement.EquallySpacedRectSide\",\"uuid\":\"8e9c2c66-c4ea-4fca-9d64-9fc616bea283\"}]},\"type\":\"ConnectorPlacement.EquallySpacedConnector\",\"uuid\":\"9d274b64-f162-4c87-866a-47fd2b4083d1\"}],\"packageUris\":[\"http://schema.mathworks.com/mf0/Connector/R2020b\"],\"version\":\"1.0\"}"
  throttle_out : Outport
  decay_mode : Outport  Port=2
  wires:
  IsNew/1 -> adaptive_throttle_contller/4(IsNew)
  adaptive_throttle_contller/2(decay_mode) -> decay_mode/1
  adaptive_throttle_contller/3(last_good_time) -> Scope1/1
  Constant/1 -> adaptive_throttle_contller/3(inc_time)
  Unit Delay/1 -> adaptive_throttle_contller/6(last_throttle)
  int_forwrd_collision_flt/1 -> adaptive_throttle_contller/2(int_forwrd_collision_flt)
  raw_throttle/1 -> adaptive_throttle_contller/1(raw_throttle)
  adaptive_throttle_contller/1(throttle_out) -> throttle_out/1, Unit Delay/1
  veh_spd/1 -> adaptive_throttle_contller/5(veh_spd)

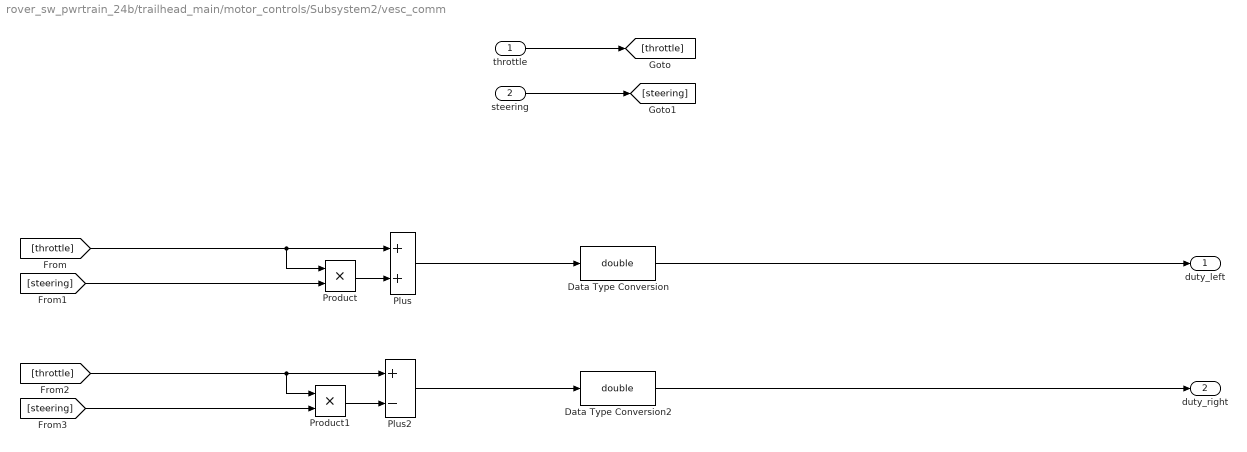
== system rover_sw_pwrtrain_24b/trailhead_main/motor_controls/Subsystem2/vesc_comm ==
  throttle : Inport
  steering : Inport  Port=2
  Data Type Conversion : DataTypeConversion  OutDataTypeStr=double  SaturateOnIntegerOverflow=off  RndMeth=Floor
  Data Type Conversion2 : DataTypeConversion  OutDataTypeStr=double  SaturateOnIntegerOverflow=off  RndMeth=Floor
  Plus : Sum
  Plus2 : Sum  Inputs=+-
  Product : Product
  Product1 : Product
  duty_left : Outport
  duty_right : Outport  Port=2
  wires:
  Product/1 -> Plus/2
  Data Type Conversion/1 -> duty_left/1
  [throttle] -> Product/1, Plus/1
  [steering] -> Product/2
  Product1/1 -> Plus2/2
  [steering] -> Product1/2
  [throttle] -> Product1/1, Plus2/1
  Data Type Conversion2/1 -> duty_right/1
  throttle/1 -> [throttle]
  steering/1 -> [steering]
  Plus/1 -> Data Type Conversion/1
  Plus2/1 -> Data Type Conversion2/1

== stateflow chart rover_sw_pwrtrain_24b/trailhead_main/arming_sequence/Chart ==
  state TRAILHEAD_UNARMED
    en:
    throttle_cmd = 0;
    steering_cmd = 0;
    mil_lamp_pwm = 1200;
  state TRAILHEAD_READY_TO_ARM
    en:
    throttle_cmd = 0;
    steering_cmd = 0;
    mil_lamp_pwm = 1300;
  state TRAILHEAD_ERROR_STATE
    en:
    throttle_cmd = 0;
    steering_cmd = 0;
    state mil_on
      du:
      mil_lamp_pwm = 1150;
    state mil_off
      du:
      mil_lamp_pwm = 500;
    (default) -> mil_on
    mil_on -> mil_off : after(3,sec)
    mil_off -> mil_on : after(1,sec)
  state TRAILHEAD_ARMED
    en:
    mil_lamp_pwm = 1500;
    du:
    steering_cmd = steering_in;
    state SLOW_ACCEL
      en:
      % Slower acceleration
      max_increase = 0.005;  % 1% per cycle
      du:
      throttle_cmd = min(throttle_in, last_throttle + max_increase);
    state FAST_DECEL
      en:
      % Faster deceleration allowed
      max_decrease = 0.05;  % 20% per cycle
      du:
      throttle_cmd = max(throttle_in, last_throttle - max_decrease);
    (default) -> SLOW_ACCEL
    SLOW_ACCEL -> FAST_DECEL : [throttle_in <= last_throttle]
    FAST_DECEL -> SLOW_ACCEL : [throttle_in > last_throttle]
  (default) -> TRAILHEAD_UNARMED
  TRAILHEAD_ARMED -> TRAILHEAD_UNARMED [order 2] : [arm_switch == OFF]
  TRAILHEAD_UNARMED -> TRAILHEAD_READY_TO_ARM : [arm_switch == OFF &&...
      | V_BATT >= 20 &&...
      | no_thottle_command == TRUE]
  TRAILHEAD_ERROR_STATE -> TRAILHEAD_UNARMED : [arm_switch == OFF]
  TRAILHEAD_READY_TO_ARM -> TRAILHEAD_ARMED : [arm_switch == ON &&...
      | V_BATT >= 20 &&...
      | abs(throttle_in) >= 0.1]
  TRAILHEAD_ARMED -> TRAILHEAD_ERROR_STATE [order 1] : after(5, sec)[V_BATT < 20]
  data: last_throttle input; steering_in input; throttle_in input; arm_switch input boolean; no_thottle_command input boolean; throttle_cmd output single; mil_lamp_pwm output int32; steering_cmd output single; OFF parameter boolean; TRUE parameter boolean; V_BATT input; ON parameter boolean; max_increase local; max_decrease local

== stateflow chart rover_sw_pwrtrain_24b/ros_publish/op_data ==
  state init
    du:
    tmr_sec = tmr_sec + .01;
    tmr_hr = tmr_sec/3600;
  (default) -> init
  data: tmr_hr output single; tmr_sec local single =0

== stateflow chart rover_sw_pwrtrain_24b/trailhead_main/motor_controls/throttle_regulation/adaptive_throttle_contller ==
  state NORMAL_OPERATION
    en:
    decay_mode = throttle_decay_mode.NORMAL;
    state SLOW_ACCEL
      en:
      % Slower acceleration
      max_increase = 0.005;  % 1% per cycle
      du:
      throttle_out = min(raw_throttle, last_throttle + max_increase);
    state FAST_DECEL
      en:
      % Faster deceleration allowed
      max_decrease = 0.05;  % 20% per cycle
      du:
      throttle_out = max(raw_throttle, last_throttle - max_decrease);
    (default) -> SLOW_ACCEL
    SLOW_ACCEL -> NORMAL_OPERATION.FAST_DECEL : [raw_throttle <= last_throttle]
  state LOSS_COMM_MONITOR
    en:
    loss_tmr = 0;
    comm_ref_throttle = last_throttle;
    du:
    loss_tmr += inc_time;
    throttle_out = last_throttle;
  state COLLISION_FLT_FAST_STOP
    en:
    collision_time = 0;
    comm_loss_time = 0;
    phase2_time = 0;
    en:
    decay_mode = throttle_decay_mode.EMERGENCY;
    du:
    collision_time = min(collision_time + inc_time, 2.5);
    state MILD
      du:
      throttle_out = max(0, last_throttle * (1 - 0.2 * collision_time));
    state SEVERE
      en: severe_time = 0;
      du:
      severe_time += inc_time;
      throttle_out = max(0, last_throttle * exp(-1.2 * severe_time));
    (default) -> MILD
    MILD -> SEVERE [order 2] : [veh_spd < .2]
    MILD -> SEVERE [order 1] : [int_forwrd_collision_flt == collision_flt.SEVERE]
  state LOST_COMM_OPERATION
    en:
    comm_loss_time = 0;
    du:
    decay_mode = throttle_decay_mode.COMM_LOSS;
    state SLOW_DECEL
      du:
      comm_loss_time += inc_time;
      throttle_out = max(0, comm_ref_throttle * (1 - 0.15 * comm_loss_time));
    state FAST_DECEL
      en:
      phase2_time = 0;
      du:
      phase2_time += inc_time;
      throttle_out = comm_ref_throttle * exp(-0.8 * phase2_time);
    (default) -> SLOW_DECEL
    SLOW_DECEL -> LOST_COMM_OPERATION.FAST_DECEL : [comm_loss_time > 20 ||...
        | veh_spd > .5]
  (default) -> (junction 41)
  (junction 42) -> NORMAL_OPERATION [order 2]
  (junction 41) -> (junction 42) [order 2]
  (junction 42) -> LOSS_COMM_MONITOR [order 1] : [IsNew == FALSE]
  (junction 41) -> COLLISION_FLT_FAST_STOP [order 1] : [int_forwrd_collision_flt ~= collision_flt.NONE]
  LOST_COMM_OPERATION -> (junction 42) [order 2] : after(10, sec)[IsNew == FALSE]
  LOSS_COMM_MONITOR -> NORMAL_OPERATION [order 2] : [IsNew == TRUE]
  NORMAL_OPERATION -> LOSS_COMM_MONITOR [order 2] : after(10,sec)[IsNew == FALSE]
  LOSS_COMM_MONITOR -> LOST_COMM_OPERATION [order 1] : [loss_tmr > 0.5]
  LOST_COMM_OPERATION -> COLLISION_FLT_FAST_STOP [order 1] : [int_forwrd_collision_flt ~= collision_flt.NONE &&...
      | IsNew == TRUE]
  COLLISION_FLT_FAST_STOP -> NORMAL_OPERATION [order 2] : [raw_throttle <= -0.1]
  COLLISION_FLT_FAST_STOP -> NORMAL_OPERATION [order 1] : after(10, sec)[int_forwrd_collision_flt == collision_flt.NONE]
  NORMAL_OPERATION -> COLLISION_FLT_FAST_STOP [order 1] : [int_forwrd_collision_flt ~= collision_flt.NONE]
  data: throttle_out output double; decay_mode output double; raw_throttle input; int_forwrd_collision_flt input; inc_time input; IsNew input; veh_spd input; dt_comm_loss local double; FALSE parameter; TRUE parameter; last_throttle input double; max_decrease local double; max_increase local double; last_good_time output double; collision_time local double; comm_loss_time local double; comm_ref_throttle local double; loss_tmr local double; phase2_time local double; severe_time local double
